simulink model "FDBlin_pend_sol"  (R2023b)
settings: Solver=ode3  StartTime=0.0  StopTime=20  FixedStep=0.01  RelTol=1e-3
values from neighbouring files (symbols this model uses):
  a = [ m ; g ; l ; d ]    [FDBlin_pend_par_sol.m]
  K = acker(A,B,p_des)    [FDBlin_pend_par_sol.m]
libraries: simulink_extras x2
settings Model: Creator=jerome  LastModifiedBy=jerome
settings ModelReferenceCC: EnableRefExpFcnMdlSchedulingChecks=on

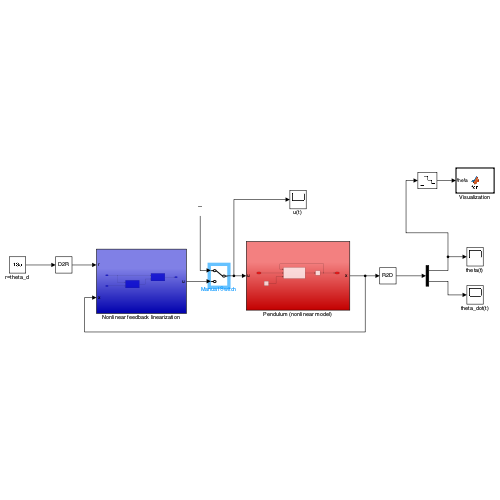
[thumbnail: Simulink's stored preview of the top-level diagram]
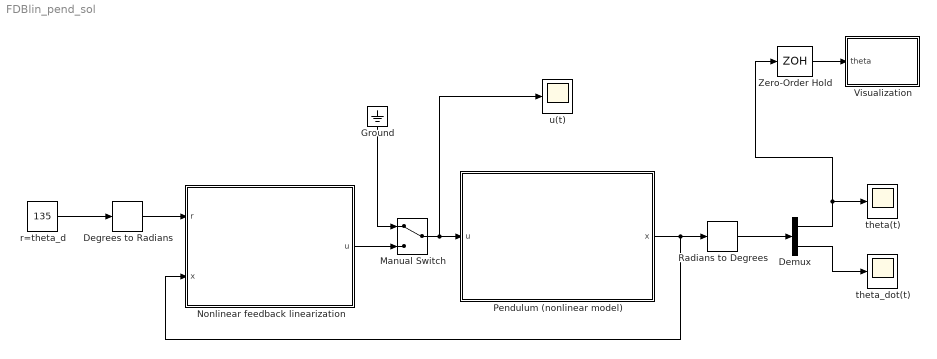
== system FDBlin_pend_sol ==
  Degrees to Radians : simulink_extras/Transformations/Degrees to Radians
  Demux : Demux  Outputs=2
  Ground : Ground
  Manual Switch : ManualSwitch
  Nonlinear feedback linearization : Subsystem
  Pendulum (nonlinear model) : Subsystem
  Radians to Degrees : simulink_extras/Transformations/Radians to Degrees
  Visualization : MATLAB Function  TreatAsAtomicUnit=on
  Zero-Order Hold : ZeroOrderHold  SampleTime=0.1
  r=theta_d : Constant  Value=135
  theta(t) : Scope
  theta_dot(t) : Scope
  u(t) : Scope
  wires:
  Pendulum (nonlinear model)/1(x) -> Nonlinear feedback linearization/2(x), Radians to Degrees/1
  Radians to Degrees/1 -> Demux/1
  Demux/2 -> theta_dot(t)/1
  r=theta_d/1 -> Degrees to Radians/1
  Degrees to Radians/1 -> Nonlinear feedback linearization/1(r)
  Zero-Order Hold/1 -> Visualization/1(theta)
  Demux/1 -> Zero-Order Hold/1, theta(t)/1
  Manual Switch/1 -> u(t)/1, Pendulum (nonlinear model)/1(u)
  Nonlinear feedback linearization/1(u) -> Manual Switch/2
  Ground/1 -> Manual Switch/1

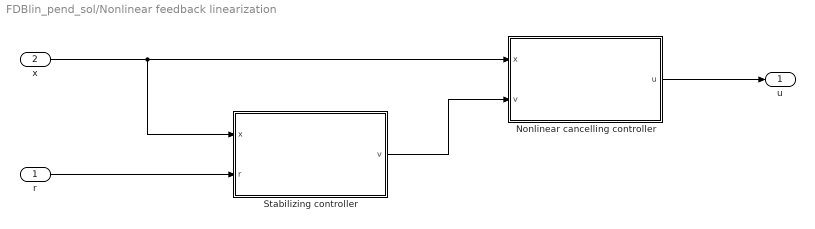
== system FDBlin_pend_sol/Nonlinear feedback linearization ==
  r : Inport
  x : Inport  Port=2
  Nonlinear cancelling controller : Subsystem
  Stabilizing controller : Subsystem
  u : Outport
  wires:
  Nonlinear cancelling controller/1(u) -> u/1
  x/1 -> Stabilizing controller/1(x), Nonlinear cancelling controller/1(x)
  Stabilizing controller/1(v) -> Nonlinear cancelling controller/2(v)
  r/1 -> Stabilizing controller/2(r)

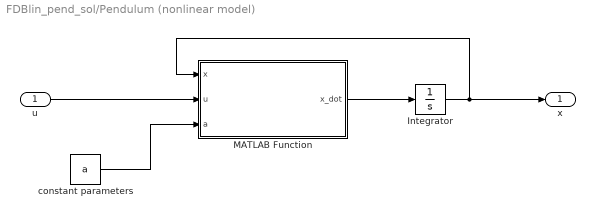
== system FDBlin_pend_sol/Pendulum (nonlinear model) ==
  u : Inport
  Integrator : Integrator  InitialCondition=[-pi/3;0]
  MATLAB Function : MATLAB Function  TreatAsAtomicUnit=on
  constant parameters : Constant  Value=a  VectorParams1D=off
  x : Outport
  wires:
  u/1 -> MATLAB Function/2(u)
  MATLAB Function/1(x_dot) -> Integrator/1
  Integrator/1 -> x/1, MATLAB Function/1(x)
  constant parameters/1 -> MATLAB Function/3(a)

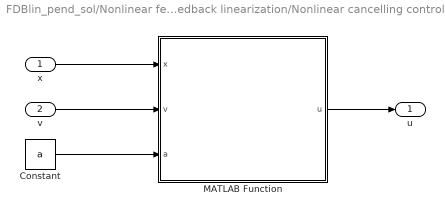
== system FDBlin_pend_sol/Nonlinear feedback linearization/Nonlinear cancelling controller ==
  x : Inport
  v : Inport  Port=2
  Constant : Constant  Value=a  VectorParams1D=off
  MATLAB Function : MATLAB Function  TreatAsAtomicUnit=on
  u : Outport
  wires:
  x/1 -> MATLAB Function/1(x)
  v/1 -> MATLAB Function/2(v)
  MATLAB Function/1(u) -> u/1
  Constant/1 -> MATLAB Function/3(a)

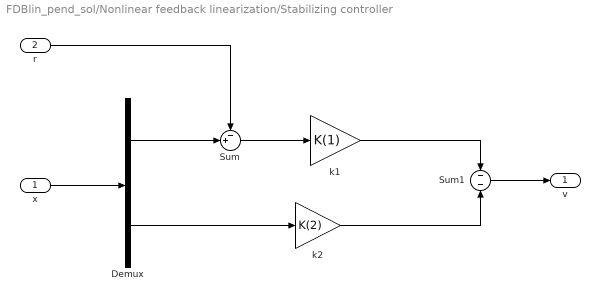
== system FDBlin_pend_sol/Nonlinear feedback linearization/Stabilizing controller ==
  x : Inport
  r : Inport  Port=2
  Demux : Demux  Outputs=2
  Sum : Sum  Inputs=-+|
  Sum1 : Sum  Inputs=--
  k1 : Gain  Gain=K(1)
  k2 : Gain  Gain=K(2)
  v : Outport
  wires:
  x/1 -> Demux/1
  Demux/1 -> Sum/2
  r/1 -> Sum/1
  Sum1/1 -> v/1
  Sum/1 -> k1/1
  k1/1 -> Sum1/1
  Demux/2 -> k2/1
  k2/1 -> Sum1/2

== matlab function FDBlin_pend_sol/Nonlinear feedback linearization/Nonlinear cancelling controller/MATLAB Function ==
  data: x input; v input; u output; a input
function u = c_lin(x,v,a)

% a is the vector of constant parameters
m = a(1);
g = a(2);
l = a(3);
d = a(4);

% cancelling controller
u = m*g*l*sin(x(1)) + d*x(2) + m*l^2*v;

== matlab function FDBlin_pend_sol/Pendulum (nonlinear model)/MATLAB Function ==
  data: x input; u input; x_dot output; a input
function x_dot = f(x,u,a)

% a is the vector of constant parameters
m = a(1);
g = a(2);
l = a(3);
d = a(4);

x_dot = [ x(2) ; 1/(m*l^2)*(-m*g*l*sin(x(1))-d*x(2)+u) ];

== matlab function FDBlin_pend_sol/Visualization ==
  data: theta input
function fcn(theta)


% body
    Ybody = [ -1 ; -1 ; 0.1 ; 0.1 ];
    Xbody = [ -0.1 ; 0.1 ; 0.1 ; -0.1 ]; 

% calculate graphical position of 2-wheel robot
      [PosXbody,PosYbody] = rot(Xbody,Ybody,deg2rad(theta));
      

% to be able to use 'fill' even though the function is not supported for code generation
% see https://se.mathworks.com/help/simulink/slref/coder.extrinsic.html
coder.extrinsic('fill'); 

% draw the body of the 2-wheel robot with the propser position and orientation
fill(PosXbody,PosYbody,'b');

axis([-1.1 1.1 -1.1 1.1]);
title('Controlled Pendulum', 'FontSize',20);
axis square;
grid on;

drawnow;



% function "rot" that rotates a graphical object
function [PosX,PosY] = rot(X,Y,angle)

dim = size(X,1);
PosX = zeros(dim,1);
PosY = zeros(dim,1);

Mrot = [ cos(angle) -sin(angle)  ;
         sin(angle)  cos(angle) ]; 

for i=1:dim
    Pos_i = Mrot * [ X(i,1) ; Y(i,1) ];
    PosX(i,1) = Pos_i(1,1);
    PosY(i,1) = Pos_i(2,1);
end
